simulink model "Worked_Example_11_3"  (R2024b)
settings: Solver=VariableStepAuto  StartTime=0.0  StopTime=6  RelTol=1e-3
settings Model: Creator=GH-X-ST  LastModifiedBy=GH-X-ST

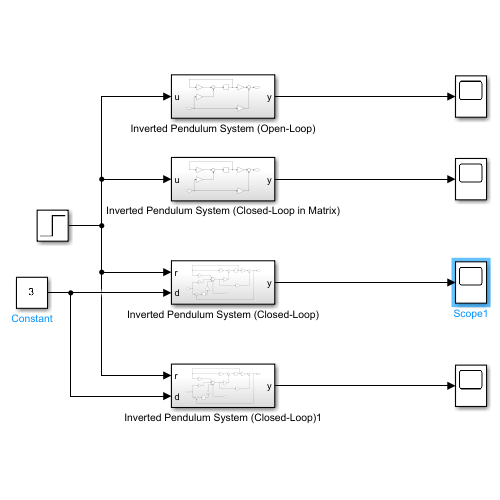
[thumbnail: Simulink's stored preview of the top-level diagram]
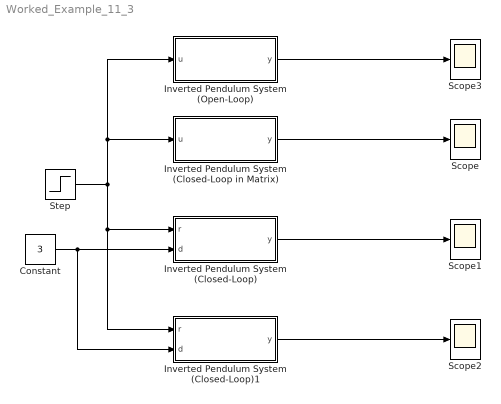
== system Worked_Example_11_3 ==
  Constant : Constant  Value=3
  Inverted Pendulum System (Closed-Loop in Matrix) : Subsystem
  Inverted Pendulum System (Closed-Loop) : Subsystem
  Inverted Pendulum System (Closed-Loop)1 : Subsystem
  Inverted Pendulum System (Open-Loop) : Subsystem
  Scope{,1..3} (4 alike) : Scope
  Step : Step  SampleTime=0
  wires:
  Step/1 -> Inverted Pendulum System (Closed-Loop)1/1(r), Inverted Pendulum System (Closed-Loop)/1(r), Inverted Pendulum System (Open-Loop)/1(u), Inverted Pendulum System (Closed-Loop in Matrix)/1(u)
  Inverted Pendulum System (Closed-Loop in Matrix)/1(y) -> Scope/1
  Inverted Pendulum System (Closed-Loop)/1(y) -> Scope1/1
  Constant/1 -> Inverted Pendulum System (Closed-Loop)1/2(d), Inverted Pendulum System (Closed-Loop)/2(d)
  Inverted Pendulum System (Closed-Loop)1/1(y) -> Scope2/1
  Inverted Pendulum System (Open-Loop)/1(y) -> Scope3/1

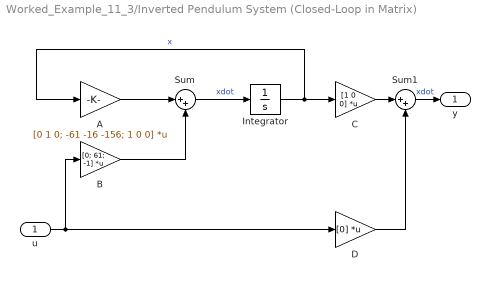
== system Worked_Example_11_3/Inverted Pendulum System (Closed-Loop in Matrix) ==
  u : Inport
  A : Gain  Gain=[0 1 0; -61 -16 -156; 1 0 0]  Multiplication=Matrix(K*u)
  B : Gain  Gain=[0; 61; -1]  Multiplication=Matrix(K*u)
  C : Gain  Gain=[1 0 0]  Multiplication=Matrix(K*u)
  D : Gain  Gain=[0]  Multiplication=Matrix(K*u)
  Integrator : Integrator  InitialCondition=[0; 0; 1]
  Sum : Sum  Inputs=|++
  Sum1 : Sum  Inputs=|++
  y : Outport
  wires:
  u/1 -> D/1, B/1
  A/1 -> Sum/1
  B/1 -> Sum/2
  Sum/1 -> Integrator/1  "xdot"
  Integrator/1 -> C/1, A/1  "x"
  C/1 -> Sum1/1
  Sum1/1 -> y/1  "xdot"
  D/1 -> Sum1/2

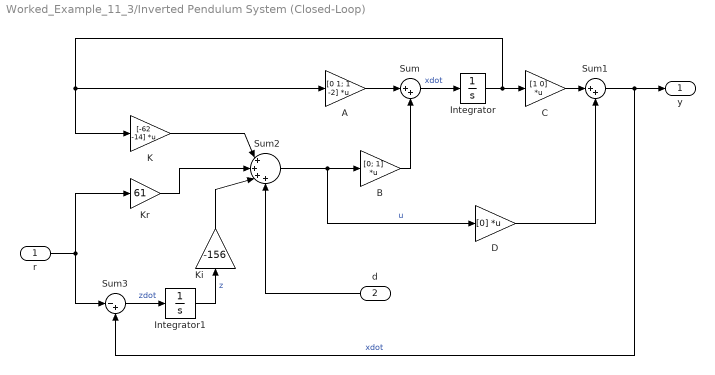
== system Worked_Example_11_3/Inverted Pendulum System (Closed-Loop) ==
  r : Inport
  d : Inport  Port=2
  A : Gain  Gain=[0 1; 1 -2]  Multiplication=Matrix(K*u)
  B : Gain  Gain=[0; 1]  Multiplication=Matrix(K*u)
  C : Gain  Gain=[1 0]  Multiplication=Matrix(K*u)
  D : Gain  Gain=[0]  Multiplication=Matrix(K*u)
  Integrator : Integrator  InitialCondition=[0;0]
  Integrator1 : Integrator  InitialCondition=1
  K : Gain  Gain=[-62 -14]  Multiplication=Matrix(K*u)
  Ki : Gain  Gain=-156
  Kr : Gain  Gain=61
  Sum : Sum  Inputs=|++
  Sum1 : Sum  Inputs=|++
  Sum2 : Sum  Inputs=|++++
  Sum3 : Sum  Inputs=|-+
  y : Outport
  wires:
  Integrator/1 -> K/1, A/1, C/1
  B/1 -> Sum/2
  r/1 -> Sum3/1, Kr/1
  D/1 -> Sum1/2
  A/1 -> Sum/1
  C/1 -> Sum1/1
  Sum1/1 -> Sum3/2, y/1  "xdot"
  Sum/1 -> Integrator/1  "xdot"
  Sum2/1 -> D/1, B/1  "u"
  Kr/1 -> Sum2/2
  Sum3/1 -> Integrator1/1  "zdot"
  Integrator1/1 -> Ki/1  "z"
  Ki/1 -> Sum2/3
  d/1 -> Sum2/4
  K/1 -> Sum2/1

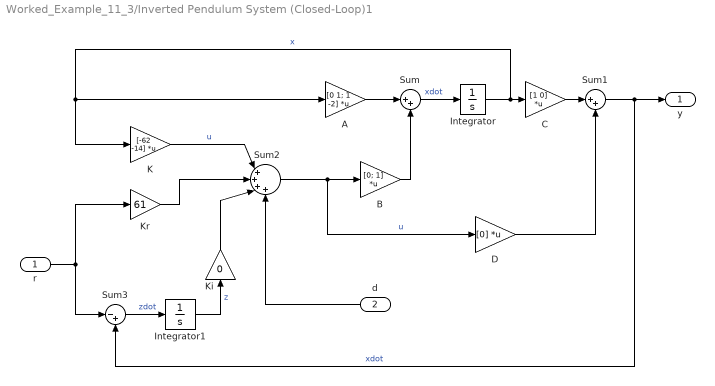
== system Worked_Example_11_3/Inverted Pendulum System (Closed-Loop)1 ==
  r : Inport
  d : Inport  Port=2
  A : Gain  Gain=[0 1; 1 -2]  Multiplication=Matrix(K*u)
  B : Gain  Gain=[0; 1]  Multiplication=Matrix(K*u)
  C : Gain  Gain=[1 0]  Multiplication=Matrix(K*u)
  D : Gain  Gain=[0]  Multiplication=Matrix(K*u)
  Integrator : Integrator  InitialCondition=[0;0]
  Integrator1 : Integrator  InitialCondition=1
  K : Gain  Gain=[-62 -14]  Multiplication=Matrix(K*u)
  Ki : Gain  Gain=0
  Kr : Gain  Gain=61
  Sum : Sum  Inputs=|++
  Sum1 : Sum  Inputs=|++
  Sum2 : Sum  Inputs=|++++
  Sum3 : Sum  Inputs=|-+
  y : Outport
  wires:
  Integrator/1 -> K/1, A/1, C/1  "x"
  B/1 -> Sum/2
  r/1 -> Sum3/1, Kr/1
  D/1 -> Sum1/2
  A/1 -> Sum/1
  C/1 -> Sum1/1
  Sum1/1 -> Sum3/2, y/1  "xdot"
  Sum/1 -> Integrator/1  "xdot"
  Sum2/1 -> D/1, B/1  "u"
  Kr/1 -> Sum2/2
  Sum3/1 -> Integrator1/1  "zdot"
  Integrator1/1 -> Ki/1  "z"
  Ki/1 -> Sum2/3
  d/1 -> Sum2/4
  K/1 -> Sum2/1  "u"

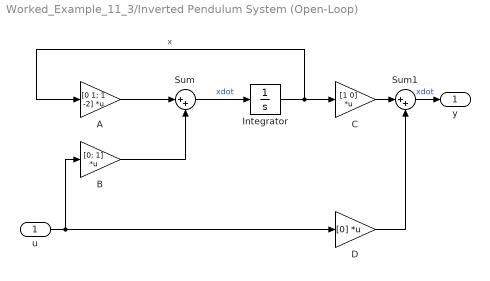
== system Worked_Example_11_3/Inverted Pendulum System (Open-Loop) ==
  u : Inport
  A : Gain  Gain=[0 1; 1 -2]  Multiplication=Matrix(K*u)
  B : Gain  Gain=[0; 1]  Multiplication=Matrix(K*u)
  C : Gain  Gain=[1 0]  Multiplication=Matrix(K*u)
  D : Gain  Gain=[0]  Multiplication=Matrix(K*u)
  Integrator : Integrator  InitialCondition=[0; 0]
  Sum : Sum  Inputs=|++
  Sum1 : Sum  Inputs=|++
  y : Outport
  wires:
  u/1 -> D/1, B/1
  A/1 -> Sum/1
  B/1 -> Sum/2
  Sum/1 -> Integrator/1  "xdot"
  Integrator/1 -> C/1, A/1  "x"
  C/1 -> Sum1/1
  Sum1/1 -> y/1  "xdot"
  D/1 -> Sum1/2
